simulink model "doubleintegrator_simple"  (R2016b)
settings: Solver=VariableStepAuto  StartTime=0.0  StopTime=10.0  RelTol=1e-3
settings Model: Creator=Guilherme  LastModifiedBy=Guilherme

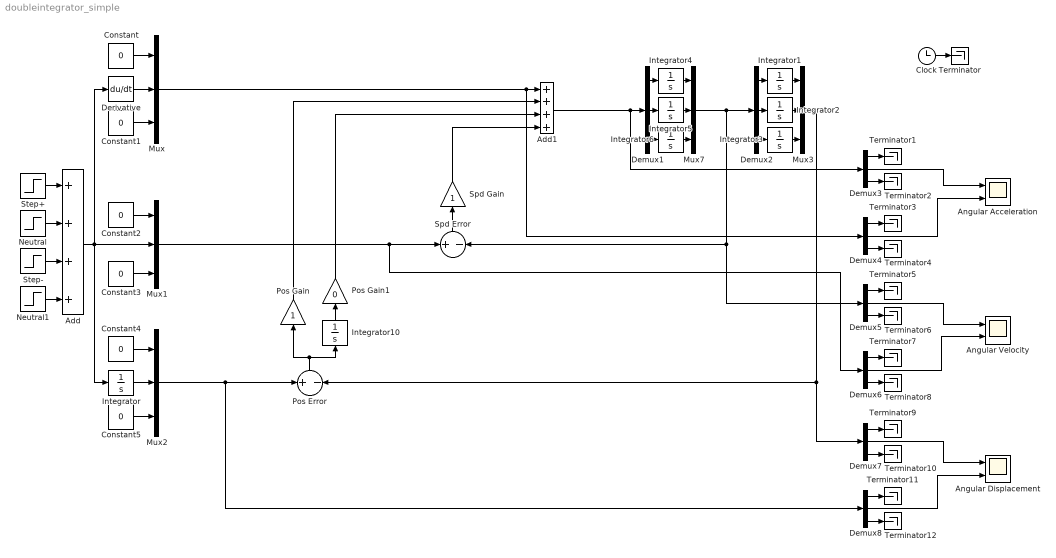
== system doubleintegrator_simple ==
  Add : Sum  Inputs=++++
  Add1 : Sum  Inputs=++++
  Angular Acceleration : Scope  NumInputPorts=2
  Angular Displacement : Scope  NumInputPorts=2
  Angular Velocity : Scope  NumInputPorts=2
  Clock : Clock
  Constant{,1..5} (6 alike) : Constant  Value=0
  Demux{1..8} (8 alike) : Demux  Outputs=3
  Derivative : Derivative
  Integrator{,1..6,10} (8 alike) : Integrator
  Mux{,1..3,7} (5 alike) : Mux  Inputs=3
  Neutral : Step  Time=2  After=-1.5  SampleTime=0
  Neutral1 : Step  Time=7  After=1.5  SampleTime=0
  Pos Error : Sum  Inputs=+-
  Pos Gain : Gain
  Pos Gain1 : Gain  Gain=0
  Spd Error : Sum  Inputs=+-
  Spd Gain : Gain
  Step+ : Step  Time=0  After=1.5  SampleTime=0
  Step- : Step  Time=5  After=-1.5  SampleTime=0
  Terminator{,1..12} (13 alike) : Terminator
  wires:
  Step+/1 -> Add/1
  Neutral/1 -> Add/2
  Step-/1 -> Add/3
  Neutral1/1 -> Add/4
  Add/1 -> Mux1/2, Integrator/1, Derivative/1
  Constant4/1 -> Mux2/1
  Integrator/1 -> Mux2/2
  Constant5/1 -> Mux2/3
  Constant1/1 -> Mux/3
  Constant/1 -> Mux/1
  Derivative/1 -> Mux/2
  Constant2/1 -> Mux1/1
  Constant3/1 -> Mux1/3
  Demux1/1 -> Integrator4/1
  Demux1/2 -> Integrator5/1
  Demux1/3 -> Integrator6/1
  Integrator4/1 -> Mux7/1
  Integrator5/1 -> Mux7/2
  Integrator6/1 -> Mux7/3
  Clock/1 -> Terminator/1
  Integrator10/1 -> Pos Gain1/1
  Mux2/1 -> Demux8/1, Pos Error/1
  Spd Error/1 -> Spd Gain/1
  Mux1/1 -> Demux6/1, Spd Error/1
  Pos Error/1 -> Integrator10/1, Pos Gain/1
  Add1/1 -> Demux3/1, Demux1/1
  Mux/1 -> Demux4/1, Add1/1
  Spd Gain/1 -> Add1/4
  Pos Gain1/1 -> Add1/3
  Pos Gain/1 -> Add1/2
  Demux2/1 -> Integrator1/1
  Demux2/2 -> Integrator2/1
  Demux2/3 -> Integrator3/1
  Integrator1/1 -> Mux3/1
  Integrator2/1 -> Mux3/2
  Integrator3/1 -> Mux3/3
  Mux7/1 -> Demux5/1, Spd Error/2, Demux2/1
  Mux3/1 -> Demux7/1, Pos Error/2
  Demux3/1 -> Terminator1/1
  Demux3/3 -> Terminator2/1
  Demux4/1 -> Terminator3/1
  Demux4/3 -> Terminator4/1
  Demux5/1 -> Terminator5/1
  Demux5/3 -> Terminator6/1
  Demux6/1 -> Terminator7/1
  Demux6/3 -> Terminator8/1
  Demux7/1 -> Terminator9/1
  Demux7/3 -> Terminator10/1
  Demux8/1 -> Terminator11/1
  Demux8/3 -> Terminator12/1
  Demux7/2 -> Angular Displacement/1
  Demux8/2 -> Angular Displacement/2
  Demux5/2 -> Angular Velocity/1
  Demux6/2 -> Angular Velocity/2
  Demux3/2 -> Angular Acceleration/1
  Demux4/2 -> Angular Acceleration/2
